simulink model "Quadrotor_eliminated_v2"  (R2020a)
settings: Solver=FixedStepAuto  StartTime=0.0  StopTime=options.T_train  FixedStep=options.dt  RelTol=1e-6
undefined symbols (not defined in the file or in its folder): options, Quad
libraries: neural x179, simulink x2
(part 7 of 10)

== system Quadrotor_eliminated_v2/NN_cex_1/Layer 2/Delays 1 ==
  "p{2}" : Inport  PortDimensions=50
      mask Display: e = 0.06;c1 = [120 230 180]/255;c2 = ([120 230 180]+0)/(256+128);c3 = ([120 230 180]+128)/(256+128);patch([0 1 1 0],[0 0 1 1],c1);patch([0 1 1 1-e 1-e 0+e],[0 0 1 1-e 0+e 0+e],c2);patch([0 0 1 1-e 0+e 0+e],[0 1 1 1-e 1-e 0+e],c3);plot([0 1 1 0 0],[0 0 1 1 0]);
  mux : Mux  Inputs=1
      mask Display: e = 0.06;c1 = [120 150 230]/255;c2 = ([120 150 230]+0)/383;c3 = ([120 150 230]+128)/383;patch([0 1 1 0],[0 0 1 1],c1);patch([0 1 1 1-e 1-e 0+e],[0 0 1 1-e 0+e 0+e],c2);patch([0 0 1 1-e 0+e 0+e],[0 1 1 1-e 1-e 0+e],c3);plot([0 1 1 0 0],[0 0 1 1 0]);disp('Mux')
  "pd{2,1}" : Outport
      mask Display: e = 0.06;c1 = [120 230 180]/255;c2 = ([120 230 180]+0)/(256+128);c3 = ([120 230 180]+128)/(256+128);patch([0 1 1 0],[0 0 1 1],c1);patch([0 1 1 1-e 1-e 0+e],[0 0 1 1-e 0+e 0+e],c2);patch([0 0 1 1-e 0+e 0+e],[0 1 1 1-e 1-e 0+e],c3);plot([0 1 1 0 0],[0 0 1 1 0]);
  wires:
  "p{2}"/1 -> mux/1
  mux/1 -> "pd{2,1}"/1

== system Quadrotor_eliminated_v2/NN_cex_1/Layer 2/LW{2,1} ==
  "ad{2,1}" : Inport  PortDimensions=50
      mask Display: e = 0.06;c1 = [120 230 180]/255;c2 = ([120 230 180]+0)/(256+128);c3 = ([120 230 180]+128)/(256+128);patch([0 1 1 0],[0 0 1 1],c1);patch([0 1 1 1-e 1-e 0+e],[0 0 1 1-e 0+e 0+e],c2);patch([0 0 1 1-e 0+e 0+e],[0 1 1 1-e 1-e 0+e],c3);plot([0 1 1 0 0],[0 0 1 1 0]);
  "IW{2,1}(1,:)'" : Constant  Value=[-0.64052430225087053639043688235688023269176483154296875;-0.67945326879490053340049371399800293147563934326171875;0.22379914523295785233614196840790100395679473876953125;-1.1886405804779995865061437143594957888126373291015625;0.09431750070984723510747471664217300713062286376953125;-1.8594326641748224471228922993759624660015106201171875;1.3635343471242842294799402225180529057979583740234375;0.0005479841448715844047512302239510972867719829082489013671875;-0.000306138059264549067250982261612080037593841552734375;-0.410664228515984053302645406802184879779815673828125;0.228212584616508618040597866638563573360443115234375;0.0303722557855780443680782099136195029132068157196044921875;-0.243137884516859414940626038514892570674419403076171875;-0.035767659341840042641624819452772499062120914459228515625;0.84026004779491281215797471304540522396564483642578125;-1.8711710850746301471048127496032975614070892333984375;-1.7103068258611464624863174321944825351238250732421875;-0.37958663757370059155249464311054907739162445068359375;3.12414617074538103480563222547061741352081298828125;-0.42708321187419751030489578624838031828403472900390625;0.93738897472706506075468269045813940465450286865234375;1.527830787786065958044900980894453823566436767578125;0.50652556608098187052036109889741055667400360107421875;1.814331905155898372328238110640086233615875244140625;-0.1284602117127590370504464090117835439741611480712890625;0.57939367711123301862841117326752282679080963134765625;-0.04046273682171565300169646661743172444403171539306640625;-0.96227523727220865001896754620247520506381988525390625;0.061823294624646508987897419729051762260496616363525390625;2.213035856114351940249207473243586719036102294921875;0.0404286989443469468863412430437165312469005584716796875;1.132012013741698464031060211709700524806976318359375;1.6605041302215770571137909428216516971588134765625;0.23123224377452300526414319392642937600612640380859375;2.52201077758148084484446371789090335369110107421875;-0.0154288540008416415194592019588526454754173755645751953125;0.63272626508026597047518180261249653995037078857421875;-0.41893867679744467569236121562425978481769561767578125;-1.5067008285940313161432868582778610289096832275390625;0.11803461310100092640507085661738528870046138763427734375;0.6030669355475397619414934524684213101863861083984375;1.723023698062699171629219563328661024570465087890625;-0.166899656535195839435203879475011490285396575927734375;-0.759281354550818576853998820297420024871826171875;-2.17639939034644580573285566060803830623626708984375;-0.447099959772296440263517069979570806026458740234375;-0.9906084050257797368743695187731646001338958740234375;-0.86527388193880894196041708710254170000553131103515625;0.77765474677443291451339746345183812081813812255859375;-0.93015712434368735817002971089095808565616607666015625]
      mask Display: e = 0.06;c1 = [120 150 230]/255;c2 = ([120 150 230]+0)/383;c3 = ([120 150 230]+128)/383;patch([0 1 1 0],[0 0 1 1],c1);patch([0 1 1 1-e 1-e 0+e],[0 0 1 1-e 0+e 0+e],c2);patch([0 0 1 1-e 0+e 0+e],[0 1 1 1-e 1-e 0+e],c3);plot([0 1 1 0 0],[0 0 1 1 0]);disp('weights');
  "IW{2,1}(2,:)'" : Constant  Value=[0.038784113531415927156320577751102973707020282745361328125;0.68340149587932630392828059484600089490413665771484375;-0.1006869434333980961593368874673615209758281707763671875;0.216715461845156387443722678654012270271778106689453125;0.6204047080493155785774206378846429288387298583984375;-0.5795805124440682742914532354916445910930633544921875;-0.5721713013251974455641857275622896850109100341796875;-0.030397184790225663386653565112283104099333286285400390625;0.1287942251430056195271589558615232817828655242919921875;-0.45209386053142031069995709913200698792934417724609375;-0.41008454425957518996170847458415664732456207275390625;-0.06289337216735195468242380911760847084224224090576171875;0.323755999414117978663085750667960382997989654541015625;-0.143803708501989924162245415573124773800373077392578125;-0.1340460391199183309840492483999696560204029083251953125;-0.2539739340422493274473936253343708813190460205078125;1.2586424777431535204641477321274578571319580078125;0.9491509203364782987222270094207488000392913818359375;-2.538804186282344499403507143142633140087127685546875;-1.488952942024968972845044845598749816417694091796875;1.9459090073693510181129795455490238964557647705078125;-0.8196679220451172920292037815670482814311981201171875;1.4755869093327314001129479947849176824092864990234375;-0.279424992039859654280320455654873512685298919677734375;-1.2893918413918097343184854253195226192474365234375;-0.7029444527448049928608497793902643024921417236328125;0.101111438350683868758750350025366060435771942138671875;-0.61468447609633958261809993928181938827037811279296875;-0.5984315204831045509337172916275449097156524658203125;0.9826045825107188047553563592373393476009368896484375;-0.33670667962498779246516278362832963466644287109375;0.51576950783507624631596399922273121774196624755859375;-1.497640433987424302131330478005111217498779296875;0.97160706638833305159863584776758216321468353271484375;-0.122788485041000094977192702572210691869258880615234375;-0.1201258763547821128980785942985676229000091552734375;-1.1609663517627504258911130818887613713741302490234375;0.57797089115618305310562163867871277034282684326171875;-0.725366805115031265671632354496978223323822021484375;-0.17505196004321221803223807000904344022274017333984375;0.99374778293694332464980334407300688326358795166015625;-0.86031542041718800373217845844919793307781219482421875;-0.9960086241980270482798687226022593677043914794921875;0.1211354491852160430997997764279716648161411285400390625;-0.65225933913535261154947875184006989002227783203125;-0.20540863167843859127259520391817204654216766357421875;-1.016696385399470603516647315700538456439971923828125;-0.104236519604504362934704886356485076248645782470703125;0.40618184640109067373714424320496618747711181640625;-0.7130520290879733824596087288227863609790802001953125]
      mask Display: e = 0.06;c1 = [120 150 230]/255;c2 = ([120 150 230]+0)/383;c3 = ([120 150 230]+128)/383;patch([0 1 1 0],[0 0 1 1],c1);patch([0 1 1 1-e 1-e 0+e],[0 0 1 1-e 0+e 0+e],c2);patch([0 0 1 1-e 0+e 0+e],[0 1 1 1-e 1-e 0+e],c3);plot([0 1 1 0 0],[0 0 1 1 0]);disp('weights');
  Mux : Mux  Inputs=2
      mask Display: e = 0.06;c1 = [120 150 230]/255;c2 = ([120 150 230]+0)/383;c3 = ([120 150 230]+128)/383;patch([0 1 1 0],[0 0 1 1],c1);patch([0 1 1 1-e 1-e 0+e],[0 0 1 1-e 0+e 0+e],c2);patch([0 0 1 1-e 0+e 0+e],[0 1 1 1-e 1-e 0+e],c3);plot([0 1 1 0 0],[0 0 1 1 0]);disp('Mux');
  dotprod1 : neural/Weight Functions/dotprod
  dotprod2 : neural/Weight Functions/dotprod
  "lz{2,1}" : Outport
      mask Display: e = 0.06;c1 = [120 230 180]/255;c2 = ([120 230 180]+0)/(256+128);c3 = ([120 230 180]+128)/(256+128);patch([0 1 1 0],[0 0 1 1],c1);patch([0 1 1 1-e 1-e 0+e],[0 0 1 1-e 0+e 0+e],c2);patch([0 0 1 1-e 0+e 0+e],[0 1 1 1-e 1-e 0+e],c3);plot([0 1 1 0 0],[0 0 1 1 0]);
  wires:
  "IW{2,1}(1,:)'"/1 -> dotprod1/1
  "ad{2,1}"/1 -> dotprod1/2, dotprod2/2
  dotprod1/1 -> Mux/1
  "IW{2,1}(2,:)'"/1 -> dotprod2/1
  dotprod2/1 -> Mux/2
  Mux/1 -> "lz{2,1}"/1

== system Quadrotor_eliminated_v2/NN_online/Layer 1/Delays 1 ==
  "p{1}" : Inport  PortDimensions=20
      mask Display: e = 0.06;c1 = [120 230 180]/255;c2 = ([120 230 180]+0)/(256+128);c3 = ([120 230 180]+128)/(256+128);patch([0 1 1 0],[0 0 1 1],c1);patch([0 1 1 1-e 1-e 0+e],[0 0 1 1-e 0+e 0+e],c2);patch([0 0 1 1-e 0+e 0+e],[0 1 1 1-e 1-e 0+e],c3);plot([0 1 1 0 0],[0 0 1 1 0]);
  mux : Mux  Inputs=1
      mask Display: e = 0.06;c1 = [120 150 230]/255;c2 = ([120 150 230]+0)/383;c3 = ([120 150 230]+128)/383;patch([0 1 1 0],[0 0 1 1],c1);patch([0 1 1 1-e 1-e 0+e],[0 0 1 1-e 0+e 0+e],c2);patch([0 0 1 1-e 0+e 0+e],[0 1 1 1-e 1-e 0+e],c3);plot([0 1 1 0 0],[0 0 1 1 0]);disp('Mux')
  "pd{1,1}" : Outport
      mask Display: e = 0.06;c1 = [120 230 180]/255;c2 = ([120 230 180]+0)/(256+128);c3 = ([120 230 180]+128)/(256+128);patch([0 1 1 0],[0 0 1 1],c1);patch([0 1 1 1-e 1-e 0+e],[0 0 1 1-e 0+e 0+e],c2);patch([0 0 1 1-e 0+e 0+e],[0 1 1 1-e 1-e 0+e],c3);plot([0 1 1 0 0],[0 0 1 1 0]);
  wires:
  "p{1}"/1 -> mux/1
  mux/1 -> "pd{1,1}"/1
